simulink model "Sim6_02_lim_current_open_close_line"  (R2019b)
settings: Solver=ode1  StartTime=0.0  StopTime=6  FixedStep=Time_Step  MaxStep=1e-4  RelTol=1e-3
undefined symbols (not defined in the file): L_1, L_2, R_1, R_2, Time_Step, Ug, VSC01_id0
libraries: powerlib x14, simulink x4, Control_Lib x4, Source_Lib x1
settings Model: Creator=Frederic_Colas  LastModifiedBy=fcolas
settings DataIOCC: ReturnWorkspaceOutputs=off
settings OptimizationCC: LifeSpan=inf
settings DebuggingCC: UnconnectedInputMsg=none  UnconnectedOutputMsg=none  UnconnectedLineMsg=none  SFExecutionAtInitializationDiag=none  ArithmeticOperatorsInVariantConditions=warning
settings HardwareCC: ProdBitPerSizeT=32  ProdBitPerPtrDiffT=32  ProdWordSize=32  ProdHWDeviceType=Specified
settings SFSimCC: SimUseLocalCustomCode=off  CustomCodeUndefinedFunction=UseInterfaceOnly
settings RTWCC: RTWUseLocalCustomCode=off
settings CodeAppCC: StateflowObjectComments=on
settings SimscapeCC: SimscapeNormalizeSystem=off

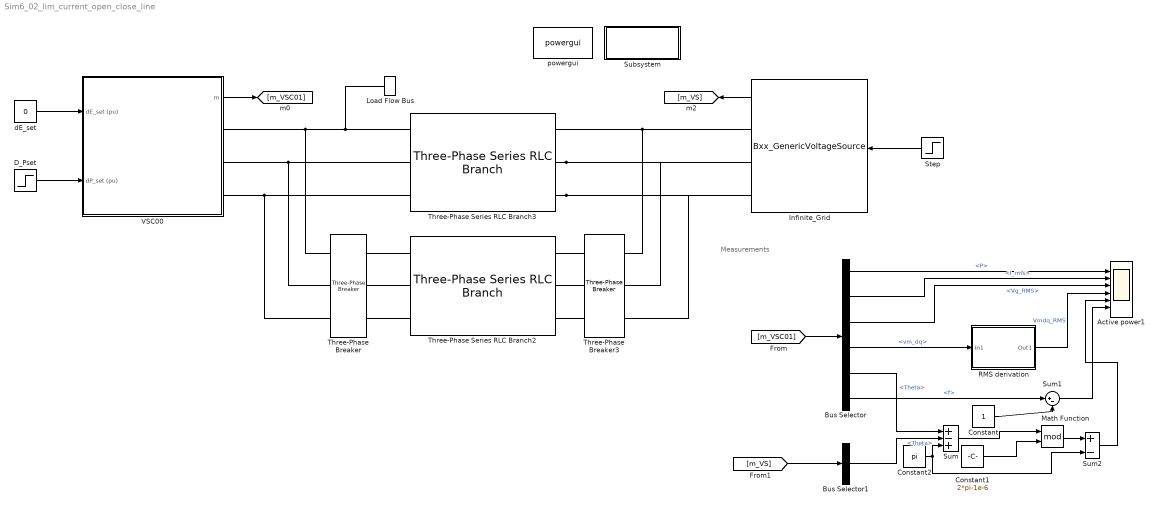
== system Sim6_02_lim_current_open_close_line ==
  note: Measurements
  Active power1 : Scope  NumInputPorts=6
  Bus Selector : BusSelector  OutputSignals=P,VI.I_rms,V.Vg_RMS,V.vm_dq,Theta.Theta,f
  Bus Selector1 : BusSelector  OutputSignals=Theta.Theta
  Constant : Constant
  Constant1 : Constant  Value=2*pi-1e-6
  Constant2 : Constant  Value=pi
  D_Pset : Step  After=0  SampleTime=0
  Infinite_Grid : Source_Lib/Bxx_GenericVoltageSource  SourceNature_str=INFINITE  fn=50  Sn=1e9  Un=Un  Time_Step=0  LFpopup=Swing  P0=-497498942.3663  Q0=24812063.8298  V0_pu=1  U0=20000  Theta0_deg=0  H_s=5  DroopOnOff=on  R_percent=4  TN=1  TD=2
      settings: SourceProductName=VSC4SPS
  Load Flow Bus : powerlib/Measurements/Load Flow Bus  LConnTagsString=a  Phases=single  Connectors=on one side  ID=BUS_1  Vbase=Un  Vref=1  Vangle=0  VLF=1.004  VLFb=1  VLFc=1  angleLF=2.855  angleLFb=0  angleLFc=0
  Math Function : Math  Operator=mod  SaturateOnIntegerOverflow=on
  RMS derivation : Subsystem
  Step : Step  Time=0.5  After=0  SampleTime=0
  Subsystem : Subsystem
      settings: OpenFcn=LoadFlow_VSC
      mask Display: color('blue'),disp('Update Loadflow')
  Sum : Sum  Inputs=+-+
  Sum1 : Sum  Inputs=|+-
  Sum2 : Sum  Inputs=+-
  Three-Phase Series RLC Branch2 : powerlib/Elements/Three-Phase Series RLC Branch  LConnTagsString=A|B|C  RConnTagsString=A|B|C  BranchType=RL  Resistance=R_2  Inductance=L_2  Capacitance=1e-6  Measurements=None
  Three-Phase Series RLC Branch3 : powerlib/Elements/Three-Phase Series RLC Branch  LConnTagsString=A|B|C  RConnTagsString=A|B|C  BranchType=RL  Resistance=R_1  Inductance=L_1  Capacitance=1e-6  Measurements=None
  Three-Phase Breaker : powerlib/Elements/Three-Phase Breaker  InitialState=closed  SwitchA=on  SwitchB=on  SwitchC=on  SwitchTimes=[1.5 4]  External=off  BreakerResistance=0.01  SnubberResistance=1e6  SnubberCapacitance=inf  Measurements=None
  Three-Phase Breaker3 : powerlib/Elements/Three-Phase Breaker  InitialState=closed  SwitchA=on  SwitchB=on  SwitchC=on  SwitchTimes=[1.5 4]  External=off  BreakerResistance=0.01  SnubberResistance=1e6  SnubberCapacitance=inf  Measurements=None
  VSC00 : Subsystem  mask(VSC){fn=50, Sn=1000e6, Pn=1000e6, Udcn=640e3, Time_Step=Time_Step, Un1=320e3, Un2=Ug, Rt_pu=0.005, Lt_pu=0.15, Lm_pu=500, Rm_pu=500, Tr_PLL=10, Val_Freq_Support=off, R_percent=4, Rv=0.09, W_TVR=60, I_max_VI_pu=1.2, DX_DR=5, Val_Mod_H=off, I_max_pu=1.25, Tr_I_max=200, Advanced=off, gainpopup=With Inertia, f_Inertia_Less=5/(2*pi), zeta_Inertia_Less=1, Param_Inertia=PI, H_GFo=5, zeta_GFo=0.7, LFpopup=PQ, P0=0.5, Q0=2.3716e-08, V0=1.0038, Theta0=2.8552}
      mask prompts: fn "Nominal Frequency (Hz)"; Sn "Nominal Apparent Power (VA)"; Pn "Nominal Power (W)"; Udcn "Nominal DC Voltage (V)"; Time_Step "Sample Time (s)"; Un1 "VSC side Nominal Ph-Ph Voltage (V)"; Un2 "Grid side Nominal Ph-Ph Voltage (V)"; Rt_pu "R (pu)"; Lt_pu "L (pu)"; Lm_pu "Rm (pu)"; Rm_pu "Lm (pu)"; Tr_PLL "Time response (ms)"; Val_Freq_Support "Frequency Support"; R_percent "Droop Gain (%)"; Rv "Damping Resistance (Rv)"; W_TVR "Dr filter"; I_max_VI_pu "Current Threshold (pu)"; Val_Mod_H "Inertia Modulation"; I_max_pu "I max (pu)"; Tr_I_max "Current Loop time response (ms)"; gainpopup "Strategy"; f_Inertia_Less "Bandwidth (Hz)"; zeta_Inertia_Less "Damping"; H_GFo "Inertia H (s)"; zeta_GFo "Damping Ratio"; P0 "Initial Active Power (pu)"; Q0 "Initial Reactive Power (pu)"; V0 "Initial Voltage (pu)"; Theta0 "Initial Angle (°)"
      mask init:
      | % Update Name of LF bus for internal purpose
      |     %NameStr = [get_param(gcb,'Name')];% '_LF'];
      |     %set_param([gcb '/Load Flow Bus'],'ID',NameStr);    
      |     
      | % Base values
      |     fb = fn;
      |     Pb = Pn;
      |     cos_phi_n = Pn/Sn;
      |     Sb = Pb/cos_phi_n;
      |     Vn1 = Un1/sqrt(3);
      |     Vb1 = Vn1;
      |     Vn2 = Un2/sqrt(3);
      |     Vb2 = Vn2;
      |     Ib1 = Sb / 3*Vb1;
      |     Ib2 = Sb / (3*Vb2);
      |     wb = 2*pi*fb;
      |   
      | % PLL derivation of the parameters
      |     wn_PLL=5/Tr_PLL;
      |     zeta_PLL = 1;
      |     Kp_PLL_pu = 2*zeta_PLL*wn_PLL/wb;
      |     Ki_PLL_pu = wn_PLL^2/wb;
      |     
      | % Grid-Forming control tuning
      |     % Inertia Less
      |     wn_Inertia_Less = 2*pi*f_Inertia_Less;
      |     Ki_Inertia_Less = Lt_pu*wn_Inertia_Less^2/wb;
      |     Kp_Inertia_Less = 2*zeta_Inertia_Less*wn_Inertia_Less*Lt_pu/wb;
      |     
      |     % With Inertia
      |     Kc = 1/(Lt_pu);
      |     kp_GFo = zeta_GFo*sqrt(2/(H_GFo*wb*Kc));
      |     kd = 2*H_GFo*kp_GFo*Kc*wb;
      | 
      | % Virtual Impedance tuning
      |     X_VI = roots([1/DX_DR^2+1 2*Lt_pu Lt_pu^2-1/I_max_VI_pu^2]);
      |     X_VI = max(X_VI);
      |     Kp_Rvi_pu = X_VI/(DX_DR*(I_max_VI_pu-1)); 
      |     
      | % Set the chosen strategy
      |     if (gainpopup == 1)
      |         Chosen_Strategy = 1;
      |     elseif (gainpopup == 2)
      |         if (Param_Inertia == 1)
      |             Chosen_Strategy = 2;
      |         elseif (Param_Inertia == 2)
      |             Chosen_Strategy = 3;
      |         end
      |     end
      |     
      | % Set the frequency droop gain
      |     R = R_percent / 100;
      | 
      | % Compute the delay compensation between control and power parts
      |     if (Time_Step == -1)
      |         Solver_Time_Step = 0;
      |     else
      |         Solver_Time_Step = Time_Step;
      |     end
      | 
      | % Compute Initial Voltage of VSC 
      | %   from steady-state output transformer model and Loadflow result
      |     
      |     %Initialize correctly the LoadFlow bus parameters connected to PCC
      |     VLF = V0;
      |     ThetaLF = Theta0;
      |     %if (LFpopup == 'PQ')
      |     %    VLF = 1;
      |     %    ThetaLF = 0;
      |     %elseif (LFpopup == 'PV')
      |     %%    VLF = V0;
      |     %    ThetaLF = 0;        
      |     %end
      |     %set_param([gcb '/Load Flow Bus'],'Vref',num2str(VLF),'Vangle',num2str(ThetaLF));
      |     
      |     R1_pu = Rt_pu/2;
      |     L1_pu = Lt_pu/2;
      |     R2_pu = Rt_pu/2;
      |     L2_pu = Lt_pu/2;
      |     X1_pu = L1_pu;
      |     X2_pu = L2_pu;
      |     Xm_pu = Lm_pu;
      |     
      |     Zm_pu = 1/(1/Rm_pu+1/(1i*Xm_pu));
      | 
      |     S0=P0+1i*Q0;
      |     I2 = conj(S0)/(V0);
      | 
      |     Vm = (R2_pu+1i*X2_pu)*I2 + V0;
      |     Im = Vm/Zm_pu;
      | 
      |     I1 = I2 + Im;
      |     V1 = (R1_pu+1i*X1_pu) * I1 + Vm;
      | 
      |     Vvsc0 = abs(V1);
      |     Theta_vsc0 = angle(V1) * 180/pi+Theta0;
      |     
      |     Va0 = Vvsc0*sqrt(2)*Vb1*sin(Theta_vsc0*pi/180);
      |     Vb0 = Vvsc0*sqrt(2)*Vb1*sin(Theta_vsc0*pi/180-2*pi/3);
      |     Vc0 = Vvsc0*sqrt(2)*Vb1*sin(Theta_vsc0*pi/180+2*pi/3);
      |     
      | % Generate string to display LF results on Mask
      |     %str_tmp = fprintf("Vvsc0 = %d, Theta_vsc0 = %d°",Vvsc0,Theta_vsc0);
      |     mo = get_param(gcb,'MaskObject');
      |     mo.getDialogControl('LF_vsc_str').Prompt = ['V0 = ', num2str(Vvsc0),' pu, Angle = ', num2str(Theta_vsc0),'°'];
      |     mo.getDialogControl('LF_pcc_str').Prompt = ['V0 = ', num2str(V0),' pu, Angle = ', num2str(Theta0),'°'];
      |     mo.getDialogControl('LF_pcc_Power_str').Prompt = ['P0 = ', num2str(P0),' pu, Q0 = ', num2str(Q0),' pu'];
      |     %set_param([gcb],'LF_str',str_tmp);
      settings: OpenFcn=|
      | NameStr = get_param(gcb,'Name');
      | open_system(gcbh, 'Mask');
      | 
      | h2AllOpenDlgs = DAStudio.ToolRoot.getOpenDialogs;
      | 
      | for i=1:length(h2AllOpenDlgs)
      |     try
      |          %disp(h2AllOpenDlgs(i).getSource.getBlock.Name);
      |         Dialog_block_name = h2AllOpenDlgs(i).getSource.getBlock.Name;
      |          %strcmp(Dialog_block_name, NameStr),
      |         if (strcmp(h2AllOpenDlgs(i).getSource.getBlock.Name, NameStr))
      |             iPos = h2AllOpenDlgs(i).position;
      |             h2AllOpenDlgs(i).position = [iPos(1)   iPos(2)   iPos(3)*1.4   iPos(4)];
      |         end
      |     end
      | end
      mask Callback Advanced:
      | % Get the mask parameter values. This is a cell
      | %   array of character vectors.
      | maskStr = get_param(gcb,'Advanced');
      | p=Simulink.Mask.get(gcb);
      | 
      | % The pop-up menu is the first mask parameter.
      | %   Check the value selected in the pop-up
      | if strcmp(maskStr,'on'),
      | 
      |     % Set the visibility of both parameters on when
      |     %   User-defined is selected in the pop-up.
      |     p.getDialogControl('TVR').Visible='on';
      |     p.getDialogControl('TVI').Visible='on';
      |     %p.getDialogControl('LC_Filter').Visible='on';
      |     p.getDialogControl('Current_Sat').Visible='on';
      |     %p.getDialogControl('Param_Strat_3').Visible='off';
      | 
      | 
      | else
      | 
      |     % Set the visibility of both parameters on when
      |     %   User-defined is selected in the pop-up.
      |     p.getDialogControl('TVR').Visible='off';
      |     p.getDialogControl('TVI').Visible='off';
      |     %p.getDialogControl('LC_Filter').Visible='off';
      |     p.getDialogControl('Current_Sat').Visible='off';
      |     %p.getDialogControl('Param_Strat_3').Visible='off';
      | 
      | end
      mask TypeOptions gainpopup: Inertia Less | With Inertia
      mask Callback gainpopup:
      | % Get the mask parameter values. This is a cell
      | %   array of character vectors.
      | maskStr = get_param(gcb,'gainpopup');
      | p=Simulink.Mask.get(gcb);
      | 
      | % The pop-up menu is the first mask parameter.
      | %   Check the value selected in the pop-up
      | if strcmp(maskStr,'Inertia Less'),
      | 
      |     % Set the visibility of both parameters on when
      |     %   User-defined is selected in the pop-up.
      |     p.getDialogControl('No_Inertia').Visible='on';
      |     p.getDialogControl('Inertia').Visible='off';
      |     %p.getDialogControl('Param_Strat_3').Visible='off';
      | 
      | 
      | elseif strcmp(maskStr,'With Inertia'),
      | 
      |     % Set the visibility of both parameters on when
      |     %   User-defined is selected in the pop-up.
      |     p.getDialogControl('No_Inertia').Visible='off';
      |     p.getDialogControl('Inertia').Visible='on';
      |     %p.getDialogControl('Param_Strat_3').Visible='off';
      | 
      | 
      |     % Turn off the visibility of the Value field
      |     %   when User-defined is not selected.
      | 
      | else
      | 
      |     % Set the visibility of both parameters on when
      |     %   User-defined is selected in the pop-up.
      |     p.getDialogControl('No_Inertia').Visible='off';
      |     p.getDialogControl('Inertia').Visible='off';
      |     %p.getDialogControl('Param_Strat_3').Visible='off';
      | 
      | end
      mask TypeOptions Param_Inertia: VSM | PI
      mask TypeOptions LFpopup: Swing | PQ | PV
      mask Callback LFpopup:
      | % Get the mask parameter values. This is a cell
      | %   array of character vectors.
      | maskStr = get_param(gcb,'LFpopup');
      | p=Simulink.Mask.get(gcb);
      | 
      | % The pop-up menu is the first mask parameter.
      | %   Check the value selected in the pop-up
      | if strcmp(maskStr,'Swing'),
      | 
      |     % Set the visibility of both parameters on when
      |     %   User-defined is selected in the pop-up.
      |     p.getParameter('P0').Visible='off';
      |     p.getParameter('Q0').Visible='off';
      |     p.getParameter('V0').Visible='on';
      |     p.getParameter('Theta0').Visible='on';
      |     set_param([gcb '/Source_For_LF'],'BusType','swing');
      | 
      | elseif strcmp(maskStr,'PQ'),
      | 
      |     % Set the visibility of both parameters on when
      |     %   User-defined is selected in the pop-up.
      |     p.getParameter('P0').Visible='on';
      |     p.getParameter('Q0').Visible='on';
      |     p.getParameter('V0').Visible='off';
      |     p.getParameter('Theta0').Visible='off';
      |     set_param([gcb '/Source_For_LF'],'BusType','PQ');
      | 
      |     % Turn off the visibility of the Value field
      |     %   when User-defined is not selected.
      | else
      | 
      |     % Set the visibility of both parameters on when
      |     %   User-defined is selected in the pop-up.
      |     p.getParameter('P0').Visible='on';
      |     p.getParameter('Q0').Visible='off';
      |     p.getParameter('V0').Visible='on';
      |     p.getParameter('Theta0').Visible='off';
      |     set_param([gcb '/Source_For_LF'],'BusType','PV');
      | 
      | end
      mask DialogControl Nominal_Param Prompt: Nominal Value
      mask DialogControl Container20 Prompt: Passive Components
      mask DialogControl Control_Param Prompt: Control Parameter
      mask DialogControl Container13 Prompt: PLL
      mask DialogControl Container14 Prompt: Frequency Support
      mask DialogControl TVR Prompt: Transient Virtual Resistor
      mask DialogControl TVI Prompt: Virtual Impedance
      mask DialogControl Current_Sat Prompt: Current Limitation
      mask DialogControl Container18 Prompt: Control Strategy
      mask DialogControl LF_Param Prompt: Loadflow
      mask DialogControl Control4 Prompt: Initial Operating Point
      mask DialogControl Container24 Prompt: VSC side
      mask DialogControl LF_vsc_str Prompt: V0 = 1.0092 pu, Angle = 7.1095°
      mask DialogControl Container25 Prompt: PCC
      mask DialogControl LF_pcc_str Prompt: V0 = 1.0038 pu, Angle = 2.8552°
      mask DialogControl LF_pcc_Power_str Prompt: P0 = 0.5 pu, Q0 = 2.3716e-08 pu
      mask DialogControl UpdateLoadflow Prompt: Update Loadflow
      mask DialogControl UpdateLoadflow Callback: LoadFlow_VSC
      mask Display:
      | x1=0.05;
      | y1=0.2;
      | %
      | plot([0.5 0.5]+x1,[0.97,0.8]-y1)
      | plot([0.5 0.32]+x1,[0.80 0.71]-y1)
      | plot([0.32 0.32]+x1,[0.80 0.52]-y1)
      | plot([0.32 0.5]+x1,[0.62 0.52]-y1)
      | plot([0.5 0.5]+x1,[0.52 0.35]-y1)
      | plot([0.45 0.5 0.43]+x1,[0.59 0.52 0.51]-y1)
      | %
      | plot([0.28 0.28]+x1,[0.74 0.58]-y1)
      | plot([0.28 0.20]+x1,[0.66 0.66]-y1)
      | %
      | plot([0.5 0.63]+x1,[0.84 0.84]-y1)
      | plot([0.63 0.63]+x1,[0.84 0.72]-y1)
      | plot([0.63 0.59]+x1,[0.72 0.65]-y1)
      | plot([0.63 0.67]+x1,[0.72 0.65]-y1)
      | plot([0.59 0.67]+x1,[0.65 0.65]-y1)
      | plot([0.63 0.63]+x1,[0.65 0.47]-y1)
      | plot([0.5 0.63]+x1,[0.47 0.47]-y1)
      | plot([0.58 0.67]+x1,[0.72 0.72]-y1)
      | %
      | color('blue')
      | text(0.3,0.10,'L-Filter GFo')
      | port_label('input',1,'dE_set (pu)');
      | port_label('input',2,'dP_set (pu)');
      | port_label('output',1,'m');
      | port_label('rconn',1,'A');
      | port_label('rconn',2,'B');
      | port_label('rconn',3,'C');
  dE_set : Constant  Value=0
  powergui : powerlib/powergui  Priority=1  SimulationMode=Discrete  SampleTime=Time_Step  frequency=60  Iterations=50  frequencyindice=50  Pbase=1000000000  ErrMax=1e-6  UnitsV=kV  UnitsW=MW  buscounter=0  FunctionMessages=off  echomessages=off  EnableUseOfTLC=off  CurrentSourceSwitches=off  DisableSnubberDevices=off  DisableRonSwitches=off  DisableVfSwitches=off  DisplayEquations=off  AutomaticDiscreteSolvers=off  SolverType=Tustin/Backward Euler (TBE)  Interpol=off  ExternalGateDelay=off  methode=off  Ts=100  x0status=blocks  SPID=on  SwTol=0  HookPort=off  NonlinearTolerance=1e-4  nMaxIteration=100  ContinueOnMaxIteration=off  RestoreLinks=warning  ResistiveCurrentMeasurement=off  Frange=[0:2:500]  Ylog=off  Xlog=on  ShowGrid=off  save=off  variable=ZData  structure=0  ZoomFFT=off  StartTime=0.0  cycles=1  DisplayStyle=1  fundamental=60  FreqAxis=off  MaxFrequency=1000  frequencyindicesteady=1  RmsSteady=1  display=off
  wires:
  dE_set/1 -> VSC00/1(dE_set (pu))
  D_Pset/1 -> VSC00/2(dP_set (pu))
  VSC00/1(m) -> [m_VSC01]
  Infinite_Grid/1 -> [m_VS]
  Step/1 -> Infinite_Grid/1
  Bus Selector/5 -> Sum/1  "<Theta>"
  Bus Selector/2 -> Active power1/2  "<I_rms>"
  RMS derivation/1(Out1) -> Active power1/4  "Vmdq_RMS"
  Sum1/1 -> Active power1/6
  Sum/1 -> Math Function/1
  Bus Selector/4 -> RMS derivation/1(In1)  "<vm_dq>"
  Bus Selector/6 -> Sum1/1  "<f>"
  Bus Selector1/1 -> Sum/2  "<Theta>"
  [m_VS] -> Bus Selector1/1
  Bus Selector/1 -> Active power1/1  "<P>"
  [m_VSC01] -> Bus Selector/1
  Bus Selector/3 -> Active power1/3  "<Vg_RMS>"
  Constant/1 -> Sum1/2
  Constant1/1 -> Math Function/2
  Math Function/1 -> Sum2/1
  Sum2/1 -> Active power1/5
  Constant2/1 -> Sum/3, Sum2/2
  connections:
  Three-Phase Breaker/LConn1 -- Three-Phase Series RLC Branch3/LConn1 -- Load Flow Bus/LConn1 -- VSC00/RConn1
  Three-Phase Series RLC Branch3/LConn3 -- VSC00/RConn3 -- Three-Phase Breaker/LConn3
  Three-Phase Series RLC Branch2/LConn2 -- Three-Phase Breaker/RConn2
  Three-Phase Series RLC Branch3/LConn2 -- VSC00/RConn2 -- Three-Phase Breaker/LConn2
  Three-Phase Series RLC Branch3/RConn2 -- Infinite_Grid/RConn2 -- Three-Phase Breaker3/RConn2
  Three-Phase Series RLC Branch2/LConn1 -- Three-Phase Breaker/RConn1
  Three-Phase Series RLC Branch2/LConn3 -- Three-Phase Breaker/RConn3
  Three-Phase Series RLC Branch3/RConn3 -- Infinite_Grid/RConn3 -- Three-Phase Breaker3/RConn3
  Three-Phase Series RLC Branch2/RConn1 -- Three-Phase Breaker3/LConn1
  Three-Phase Series RLC Branch2/RConn3 -- Three-Phase Breaker3/LConn3
  Three-Phase Series RLC Branch2/RConn2 -- Three-Phase Breaker3/LConn2
  Three-Phase Series RLC Branch3/RConn1 -- Three-Phase Breaker3/RConn1 -- Infinite_Grid/RConn1

== system Sim6_02_lim_current_open_close_line/RMS derivation ==
  In1 : Inport
  Demux : Demux  Outputs=2
  Sqrt : Sqrt  SaturateOnIntegerOverflow=on
  Square : Math  Operator=square  SaturateOnIntegerOverflow=on
  Square1 : Math  Operator=square  SaturateOnIntegerOverflow=on
  Sum : Sum
  Out1 : Outport
  wires:
  Square1/1 -> Sum/2
  Sum/1 -> Sqrt/1
  Sqrt/1 -> Out1/1
  Demux/1 -> Square/1
  Square/1 -> Sum/1
  Demux/2 -> Square1/1
  In1/1 -> Demux/1

== system Sim6_02_lim_current_open_close_line/Subsystem ==

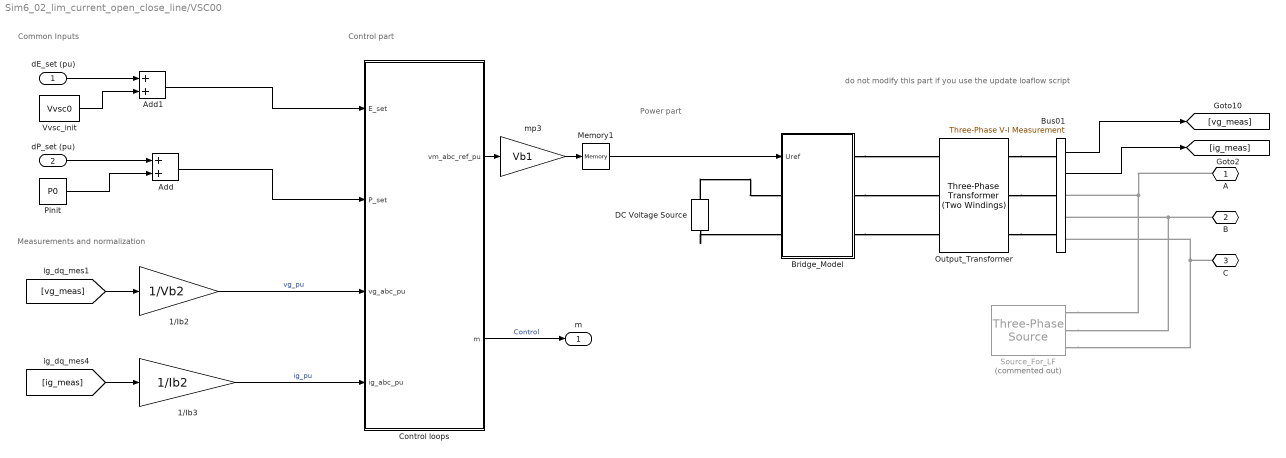
== system Sim6_02_lim_current_open_close_line/VSC00 ==
  note: do not modify this part if you use the update loaflow script
  note: Common Inputs
  note: Power part
  note: Measurements and normalization
  note: Control part
  dE_set (pu) : Inport
  dP_set (pu) : Inport  Port=2
  1/Ib2 : Gain  Gain=1/Vb2
  1/Ib3 : Gain  Gain=1/Ib2
  Add : Sum
  Add1 : Sum
  Bridge_Model : Subsystem
  Bus01 : powerlib/Measurements/Three-Phase V-I Measurement  VoltageMeasurement=phase-to-ground  SetLabelV=off  LabelV=Vabc  Vpu=off  VpuLL=off  CurrentMeasurement=yes  SetLabelI=off  LabelI=Iabc  Ipu=off  Pbase=100e6  Vbase=500e3  OutputType=Complex  PhasorSimulation=off  PSBequivalent=0
  Control loops : Subsystem
  DC Voltage Source : powerlib/Electrical Sources/DC Voltage Source  Amplitude=Udcn  Measurements=Voltage
  Memory1 : Memory  InitialCondition=[Va0 Vb0 Vc0]
  Output_Transformer : powerlib/Elements/Three-Phase Transformer (Two Windings)  Winding1Connection=Yg  Winding2Connection=Yg  CoreType=Three single-phase transformers  SetSaturation=off  Hysteresis=off  DataFile='hysteresis'  SetInitialFlux=off  Measurements=None  UNITS=pu  NominalPower=[Sn , fb]  Winding1=[Un1 , Rt_pu/2 , Lt_pu/2]  Winding2=[Un2 , Rt_pu/2 , Lt_pu/2]  Rm=Rm_pu  Lm=Lm_pu  L0=0.5  Saturation=[ 0,0 ; 0.0024,1.2 ; 1.0,1.52 ]  InitialFluxes=[ 0.8 , -0.8 , 0.7 ]  BreakLoop=off  DiscreteSolver=Trapezoidal iterative  DataType=off  TransfoNumber=1
  Pinit : Constant  Value=P0
  Source_For_LF : powerlib/Electrical Sources/Three-Phase Source  Commented=on  InternalConnection=Yg  VoltagePhases=off  Voltage=(400000)*1.00378  PhaseAngle=2.8552  Voltage_phases=[25e3 25e3 25e3]/sqrt(3)  PhaseAngles_phases=[0 -120 +120]  Frequency=fb  NonIdealSource=off  SpecifyImpedance=off  Resistance=0  Inductance=0  ShortCircuitLevel=100e6  BaseVoltage=Un  XRratio=7  BusType=PQ  Pref=P0*Sb  Qref=Q0*Sb  Prefabc=[10e3, 10e3, 10e3]  Qrefabc=[0, 0, 0]  Qmin=-inf  Qmax=inf
  Vvsc_init : Constant  Value=Vvsc0
  mp3 : Gain  Gain=Vb1
  A : PMIOPort  Side=Right
  B : PMIOPort  Port=2  Side=Right
  C : PMIOPort  Port=3  Side=Right
  m : Outport  VectorParamsAs1DForOutWhenUnconnected=off
  wires:
  Add/1 -> Control loops/2(P_set)
  Control loops/2(m) -> m/1  "Control"
  mp3/1 -> Memory1/1
  1/Ib3/1 -> Control loops/4(ig_abc_pu)  "ig_pu"
  1/Ib2/1 -> Control loops/3(vg_abc_pu)  "vg_pu"
  [vg_meas] -> 1/Ib2/1
  Control loops/1(vm_abc_ref_pu) -> mp3/1
  Add1/1 -> Control loops/1(E_set)
  Memory1/1 -> Bridge_Model/1(Uref)
  dP_set (pu)/1 -> Add/1
  Pinit/1 -> Add/2
  Vvsc_init/1 -> Add1/2
  Bus01/1 -> [vg_meas]
  dE_set (pu)/1 -> Add1/1
  Bus01/2 -> [ig_meas]
  [ig_meas] -> 1/Ib3/1
  connections:
  DC Voltage Source/LConn1 -- Bridge_Model/LConn2
  Output_Transformer/RConn1 -- Bus01/LConn1
  Output_Transformer/RConn2 -- Bus01/LConn2
  DC Voltage Source/RConn1 -- Bridge_Model/LConn1
  Output_Transformer/RConn3 -- Bus01/LConn3
  Source_For_LF/RConn2 -- B/RConn1 -- Bus01/RConn2
  Bridge_Model/RConn1 -- Output_Transformer/LConn1
  Bridge_Model/RConn2 -- Output_Transformer/LConn2
  Bridge_Model/RConn3 -- Output_Transformer/LConn3
  Source_For_LF/RConn1 -- A/RConn1 -- Bus01/RConn1
  Source_For_LF/RConn3 -- C/RConn1 -- Bus01/RConn3

== system Sim6_02_lim_current_open_close_line/VSC00/Bridge_Model ==
  Uref : Inport
  Constant : Constant
  Memory : Memory
  NOT1 : Logic  Operator=NOT  IconShape=distinctive  AllPortsSameDT=off  OutDataTypeStr=boolean
  Saturation : Saturate  UpperLimit=1  LowerLimit=-1
  Three-Phase Breaker1 : powerlib/Elements/Three-Phase Breaker  InitialState=closed  SwitchA=on  SwitchB=on  SwitchC=on  SwitchTimes="[4/60  10/60]"  External=on  BreakerResistance=0.001  SnubberResistance=1e6  SnubberCapacitance=inf  Measurements=None
  Three-Phase Breaker2 : powerlib/Elements/Three-Phase Breaker  InitialState=open  SwitchA=on  SwitchB=on  SwitchC=on  SwitchTimes="[4/60  10/60]"  External=on  BreakerResistance=0.001  SnubberResistance=1e6  SnubberCapacitance=inf  Measurements=None
  Three-Phase Source : powerlib/Electrical Sources/Three-Phase Source  InternalConnection=Yg  VoltagePhases=off  Voltage=Vvsc0*Un1  PhaseAngle=Theta_vsc0  Voltage_phases=[25e3 25e3 25e3]/sqrt(3)  PhaseAngles_phases=[0 -120 +120]  Frequency=fb  NonIdealSource=off  SpecifyImpedance=off  Resistance=0  Inductance=0  ShortCircuitLevel=100e6  BaseVoltage=VSC01_Un1  XRratio=7  BusType=swing  Pref=0.3  Qref=0  Prefabc=[10e3, 10e3, 10e3]  Qrefabc=[0, 0, 0]  Qmin=-Inf  Qmax=Inf
  Universal Bridge : powerlib/Power Electronics/Universal Bridge  Arms=3  SnubberResistance=1e5  SnubberCapacitance=inf  Device=Average-model based VSC  Ron=1e-3  Lon=0  ForwardVoltages="[  0  0  ]"  ForwardVoltage=0  GTOparameters=[ 10e-6 , 20e-6 ]  IGBTparameters=[ 1e-6 , 2e-6 ]  Measurements=None  Measurements_2=None  converterType=Rectifier
  mp3 : Gain  Gain=2/Udcn
  PhA : PMIOPort  Side=Right
  PhB : PMIOPort  Port=2  Side=Right
  PhC : PMIOPort  Port=3  Side=Right
  Vdc+ : PMIOPort  Port=4  Side=Left
  Vdc- : PMIOPort  Port=5  Side=Left
  wires:
  Saturation/1 -> Universal Bridge/1
  Constant/1 -> Memory/1
  NOT1/1 -> Three-Phase Breaker1/1
  Memory/1 -> NOT1/1, Three-Phase Breaker2/1
  mp3/1 -> Saturation/1
  Uref/1 -> mp3/1
  connections:
  Three-Phase Breaker2/LConn1 -- Three-Phase Breaker1/LConn1 -- PhA/RConn1
  Three-Phase Breaker2/LConn2 -- Three-Phase Breaker1/LConn2 -- PhB/RConn1
  Three-Phase Breaker2/LConn3 -- Three-Phase Breaker1/LConn3 -- PhC/RConn1
  Three-Phase Breaker2/RConn1 -- Universal Bridge/LConn1
  Three-Phase Breaker2/RConn2 -- Universal Bridge/LConn2
  Three-Phase Breaker2/RConn3 -- Universal Bridge/LConn3
  Three-Phase Source/RConn1 -- Three-Phase Breaker1/RConn1
  Three-Phase Source/RConn2 -- Three-Phase Breaker1/RConn2
  Three-Phase Source/RConn3 -- Three-Phase Breaker1/RConn3
  Universal Bridge/RConn1 -- Vdc+/RConn1
  Universal Bridge/RConn2 -- Vdc-/RConn1

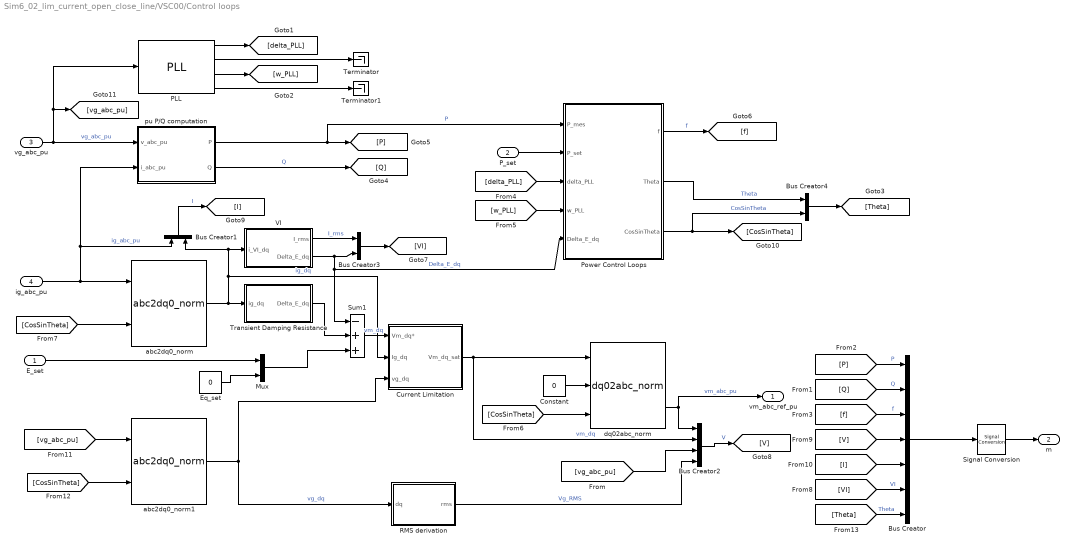
== system Sim6_02_lim_current_open_close_line/VSC00/Control loops ==
  E_set : Inport
  P_set : Inport  Port=2
  vg_abc_pu : Inport  Port=3
  ig_abc_pu : Inport  Port=4
  " pu P/Q computation" : Subsystem  DialogController=POWERSYS.PowerSysDialog
  Bus Creator : BusCreator  Inputs=7
  Bus Creator1 : BusCreator  Inputs=2
  Bus Creator2 : BusCreator  Inputs=4
  Bus Creator3 : BusCreator  Inputs=2
  Bus Creator4 : BusCreator  Inputs=2
  Constant : Constant  Value=0
  Current Limitation : Subsystem
  Eq_set : Constant  Value=0
  Mux : Mux  Inputs=2
  PLL : Control_Lib/PLL  fb=fb  Tr_PLL=Tr_PLL  Theta0=Theta0
      settings: SourceProductName=VSC_Lib
  Power Control Loops : Subsystem
  RMS derivation : Subsystem
  Signal Conversion : SignalConversion  OverrideOpt=off
  Sum1 : Sum  Inputs=-++
  Terminator : Terminator
  Terminator1 : Terminator
  Transient Damping Resistance : Subsystem
  VI : Subsystem
  abc2dq0_norm : Control_Lib/abc2dq0_norm  referenceAxisMode=Reference axis at 90 degrees behind phase_a  baseUpdateGain=1/sqrt(3)
      settings: SourceProductName=VSC_Lib
  abc2dq0_norm1 : Control_Lib/abc2dq0_norm  referenceAxisMode=Reference axis at 90 degrees behind phase_a  baseUpdateGain=1/sqrt(3)
      settings: SourceProductName=VSC_Lib
  dq02abc_norm : Control_Lib/dq02abc_norm  referenceAxisMode=Reference axis at 90 degrees behind phase_a  baseUpdateGain=sqrt(3)
      settings: SourceProductName=VSC_Lib
  vm_abc_ref_pu : Outport  VectorParamsAs1DForOutWhenUnconnected=off
  m : Outport  Port=2  VectorParamsAs1DForOutWhenUnconnected=off
  wires:
  [Theta] -> Bus Creator/7  "Theta"
  Bus Creator4/1 -> [Theta]
  RMS derivation/1(rms) -> Bus Creator2/4  "Vg_RMS"
  [vg_abc_pu] -> Bus Creator2/3
  Bus Creator3/1 -> [VI]
  PLL/4 -> Terminator1/1
  PLL/2 -> Terminator/1
  PLL/1 -> [delta_PLL]
  Constant/1 -> dq02abc_norm/2
  Power Control Loops/3(CosSinTheta) -> [CosSinTheta], Bus Creator4/2  "CosSinTheta"
  PLL/3 -> [w_PLL]
  [I] -> Bus Creator/5
  Bus Creator1/1 -> [I]  "I"
  Bus Creator/1 -> Signal Conversion/1
  [VI] -> Bus Creator/6  "VI"
  [V] -> Bus Creator/4
  Bus Creator2/1 -> [V]  "V"
  Eq_set/1 -> Mux/2
  Mux/1 -> Sum1/3
  VI/1(I_rms) -> Bus Creator3/1  "I_rms"
  Transient Damping Resistance/1("Delta_E_dq ") -> Sum1/2
  VI/2(Delta_E_dq) -> Bus Creator3/2, Sum1/1, Power Control Loops/5(Delta_E_dq)  "Delta_E_dq"
  [CosSinTheta] -> abc2dq0_norm/2
  [CosSinTheta] -> dq02abc_norm/3
  Power Control Loops/2(Theta) -> Bus Creator4/1  "Theta"
  abc2dq0_norm/2 -> Bus Creator1/2, VI/1(i_VI_dq), Current Limitation/2(Ig_dq), Transient Damping Resistance/1(ig_dq)  "ig_dq"
  ig_abc_pu/1 -> abc2dq0_norm/1, " pu P/Q computation"/2(i_abc_pu), Bus Creator1/1  "ig_abc_pu"
  " pu P/Q computation"/1(P) -> [P], Power Control Loops/1(P_mes)  "P"
  vg_abc_pu/1 -> PLL/1, [vg_abc_pu], " pu P/Q computation"/1(v_abc_pu)  "vg_abc_pu"
  Power Control Loops/1(f) -> [f]  "f"
  [w_PLL] -> Power Control Loops/4(w_PLL)
  P_set/1 -> Power Control Loops/2(P_set)
  [delta_PLL] -> Power Control Loops/3(delta_PLL)
  Current Limitation/1(Vm_dq_sat) -> dq02abc_norm/1, Bus Creator2/2  "vm_dq"
  " pu P/Q computation"/2(Q) -> [Q]  "Q"
  E_set/1 -> Mux/1
  dq02abc_norm/2 -> Bus Creator2/1, vm_abc_ref_pu/1  "vm_abc_pu"
  [f] -> Bus Creator/3  "f"
  [Q] -> Bus Creator/2  "Q"
  [P] -> Bus Creator/1  "P"
  Signal Conversion/1 -> m/1
  Sum1/1 -> Current Limitation/1(Vm_dq*)  "vm_dq"
  [vg_abc_pu] -> abc2dq0_norm1/1
  [CosSinTheta] -> abc2dq0_norm1/2
  abc2dq0_norm1/2 -> Current Limitation/3(vg_dq), RMS derivation/1(dq)  "vg_dq"

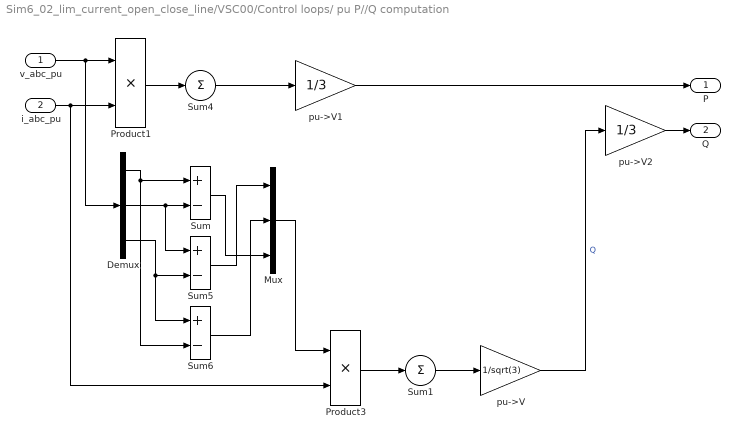
== system Sim6_02_lim_current_open_close_line/VSC00/Control loops/ pu P//Q computation ==
  v_abc_pu : Inport  PortDimensions=3
  i_abc_pu : Inport  Port=2  PortDimensions=3
  Demux : Demux  Outputs=3
      settings: DisplayOption=none
  Mux : Mux  Inputs=3
  Product1 : Product  InputSameDT=on  SaturateOnIntegerOverflow=on  OutDataTypeStr=Inherit: Same as first input
  Product3 : Product  InputSameDT=on  SaturateOnIntegerOverflow=on  OutDataTypeStr=Inherit: Same as first input
  Sum : Sum  Inputs=+-  InputSameDT=on  SaturateOnIntegerOverflow=on  OutDataTypeStr=Inherit: Same as first input
  Sum1 : Sum  Inputs=1  InputSameDT=on  SaturateOnIntegerOverflow=on  OutDataTypeStr=Inherit: Same as first input
  Sum4 : Sum  Inputs=1  InputSameDT=on  SaturateOnIntegerOverflow=on  OutDataTypeStr=Inherit: Same as first input
  Sum5 : Sum  Inputs=+-  InputSameDT=on  SaturateOnIntegerOverflow=on  OutDataTypeStr=Inherit: Same as first input
  Sum6 : Sum  Inputs=+-  InputSameDT=on  SaturateOnIntegerOverflow=on  OutDataTypeStr=Inherit: Same as first input
  pu->V : Gain  Gain=1/sqrt(3)  SaturateOnIntegerOverflow=on  OutDataTypeStr=Inherit: Same as input  ParamDataTypeStr=Inherit: Same as input
  pu->V1 : Gain  Gain=1/3  SaturateOnIntegerOverflow=on  OutDataTypeStr=Inherit: Same as input  ParamDataTypeStr=Inherit: Same as input
  pu->V2 : Gain  Gain=1/3  SaturateOnIntegerOverflow=on  OutDataTypeStr=Inherit: Same as input  ParamDataTypeStr=Inherit: Same as input
  P : Outport  VectorParamsAs1DForOutWhenUnconnected=off
  Q : Outport  Port=2  VectorParamsAs1DForOutWhenUnconnected=off
  wires:
  pu->V2/1 -> Q/1
  pu->V1/1 -> P/1
  Sum1/1 -> pu->V/1
  Product3/1 -> Sum1/1
  Product1/1 -> Sum4/1
  v_abc_pu/1 -> Product1/1, Demux/1
  i_abc_pu/1 -> Product1/2, Product3/2
  Sum4/1 -> pu->V1/1
  Demux/1 -> Sum/1, Sum6/2
  Demux/2 -> Sum/2, Sum5/1
  Demux/3 -> Sum5/2, Sum6/1
  Sum/1 -> Mux/3
  Sum5/1 -> Mux/1
  Sum6/1 -> Mux/2
  Mux/1 -> Product3/1
  pu->V/1 -> pu->V2/1  "Q"

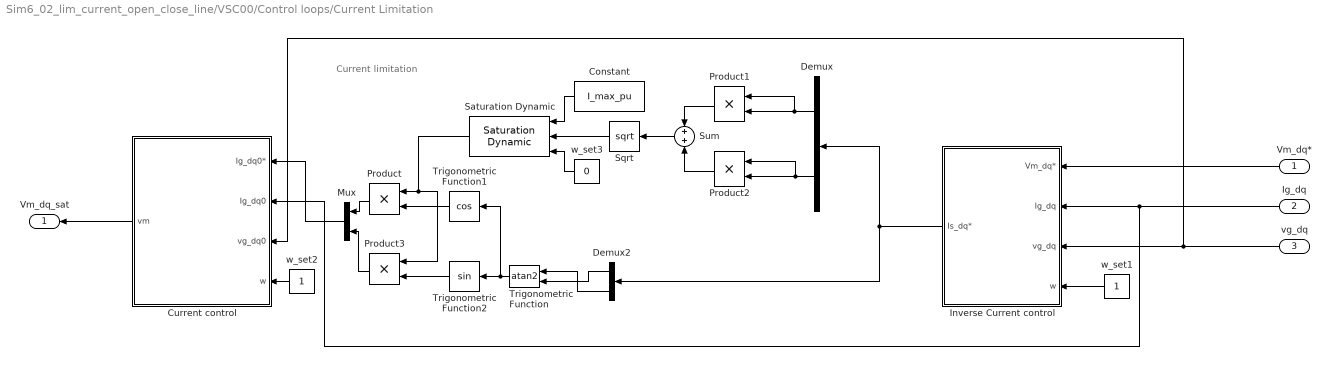
== system Sim6_02_lim_current_open_close_line/VSC00/Control loops/Current Limitation ==
  note: Current limitation
  Vm_dq* : Inport
  Ig_dq : Inport  Port=2
  vg_dq : Inport  Port=3
  Constant : Constant  Value=I_max_pu
  Current control : Subsystem
  Demux : Demux  Outputs=2
  Demux2 : Demux  Outputs=2
  Inverse Current control : Subsystem
  Mux : Mux  Inputs=2
  Product{,1..3} (4 alike) : Product
  Saturation Dynamic : simulink/Discontinuities/Saturation Dynamic  OutMin=[]  OutMax=[]  OutDataTypeStr=Inherit: Same as second input  OutDataType=fixdt(1, 16)  OutScaling=2^-10  DoSatur=off
  Sqrt : Sqrt  SaturateOnIntegerOverflow=on
  Sum : Sum
  Trigonometric Function : Trigonometry  Operator=atan2  NumberOfIterations=5  OutputSignalType=real
  Trigonometric Function1 : Trigonometry  Operator=cos
  Trigonometric Function2 : Trigonometry
  w_set1 : Constant
  w_set2 : Constant
  w_set3 : Constant  Value=0
  Vm_dq_sat : Outport  VectorParamsAs1DForOutWhenUnconnected=off
  wires:
  w_set3/1 -> Saturation Dynamic/3
  Constant/1 -> Saturation Dynamic/1
  Mux/1 -> Current control/1(Ig_dq0*)
  Product/1 -> Mux/1
  Demux/1 -> Product1/1, Product1/2
  Demux/2 -> Product2/1, Product2/2
  Trigonometric Function2/1 -> Product3/2
  Product2/1 -> Sum/2
  Trigonometric Function1/1 -> Product/2
  Demux2/1 -> Trigonometric Function/2
  Trigonometric Function/1 -> Trigonometric Function2/1, Trigonometric Function1/1
  Saturation Dynamic/1 -> Product/1, Product3/1
  Product1/1 -> Sum/1
  Sqrt/1 -> Saturation Dynamic/2
  Demux2/2 -> Trigonometric Function/1
  Inverse Current control/1(Is_dq*) -> Demux2/1, Demux/1
  Sum/1 -> Sqrt/1
  Product3/1 -> Mux/2
  Ig_dq/1 -> Inverse Current control/2(Ig_dq), Current control/2(Ig_dq0)
  w_set1/1 -> Inverse Current control/4(w)
  w_set2/1 -> Current control/4(w)
  vg_dq/1 -> Current control/3(vg_dq0), Inverse Current control/3(vg_dq)
  Vm_dq*/1 -> Inverse Current control/1(Vm_dq*)
  Current control/1(vm) -> Vm_dq_sat/1

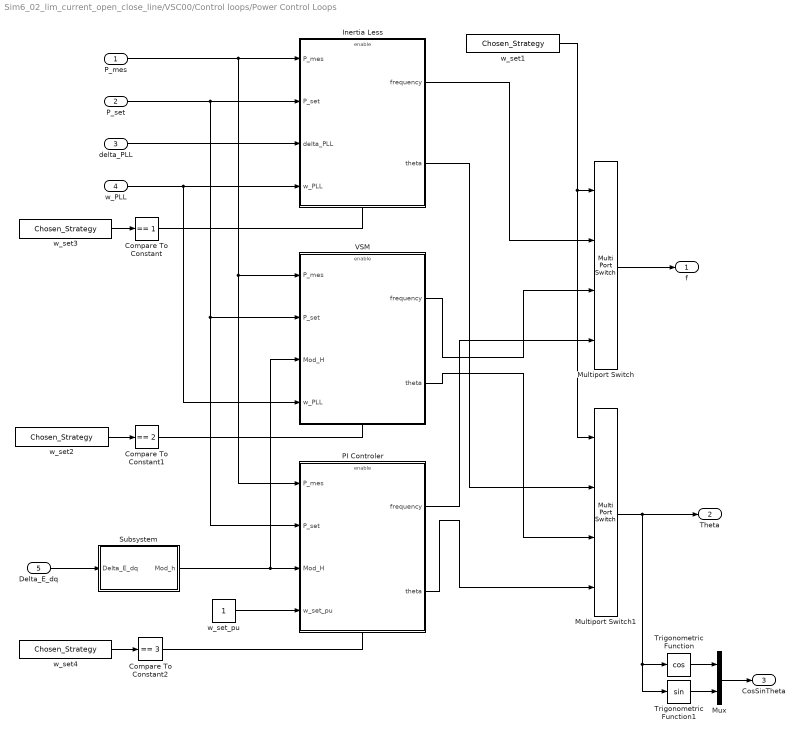
== system Sim6_02_lim_current_open_close_line/VSC00/Control loops/Power Control Loops ==
  P_mes : Inport
  P_set : Inport  Port=2
  delta_PLL : Inport  Port=3
  w_PLL : Inport  Port=4
  Delta_E_dq : Inport  Port=5
  Compare To Constant : simulink/Logic and Bit Operations/Compare To Constant  relop===  const=1  OutDataTypeStr=boolean
  Compare To Constant1 : simulink/Logic and Bit Operations/Compare To Constant  relop===  const=2  OutDataTypeStr=boolean
  Compare To Constant2 : simulink/Logic and Bit Operations/Compare To Constant  relop===  const=3  OutDataTypeStr=boolean
  Inertia Less : Subsystem
  Multiport Switch : MultiPortSwitch
  Multiport Switch1 : MultiPortSwitch
  Mux : Mux  Inputs=[1 1]
  PI Controler : Subsystem
  Subsystem : Subsystem
  Trigonometric Function : Trigonometry  Operator=cos
  Trigonometric Function1 : Trigonometry
  VSM : Subsystem
  w_set{1..4} (4 alike) : Constant  Value=Chosen_Strategy
  w_set_pu : Constant
  f : Outport  PortDimensions=1  VectorParamsAs1DForOutWhenUnconnected=off
  Theta : Outport  Port=2  VectorParamsAs1DForOutWhenUnconnected=off
  CosSinTheta : Outport  Port=3  PortDimensions=2  VectorParamsAs1DForOutWhenUnconnected=off
  wires:
  Subsystem/1(Mod_h) -> PI Controler/3(Mod_H), VSM/3(Mod_H)
  Delta_E_dq/1 -> Subsystem/1(Delta_E_dq)
  Multiport Switch1/1 -> Trigonometric Function1/1, Trigonometric Function/1, Theta/1
  Trigonometric Function1/1 -> Mux/2
  Mux/1 -> CosSinTheta/1
  Trigonometric Function/1 -> Mux/1
  Compare To Constant2/1 -> PI Controler/Enable
  Compare To Constant1/1 -> VSM/Enable
  Compare To Constant/1 -> Inertia Less/Enable
  w_set4/1 -> Compare To Constant2/1
  w_set2/1 -> Compare To Constant1/1
  w_set3/1 -> Compare To Constant/1
  Inertia Less/1(frequency) -> Multiport Switch/2
  Multiport Switch/1 -> f/1
  Inertia Less/2(theta) -> Multiport Switch1/2
  VSM/2(theta) -> Multiport Switch1/3
  w_set1/1 -> Multiport Switch/1, Multiport Switch1/1
  VSM/1(frequency) -> Multiport Switch/3
  PI Controler/1(frequency) -> Multiport Switch/4
  PI Controler/2(theta) -> Multiport Switch1/4
  w_set_pu/1 -> PI Controler/4(w_set_pu)
  w_PLL/1 -> Inertia Less/4(w_PLL), VSM/4(w_PLL)
  delta_PLL/1 -> Inertia Less/3(delta_PLL)
  P_set/1 -> Inertia Less/2(P_set), VSM/2(P_set), PI Controler/2(P_set)
  P_mes/1 -> Inertia Less/1(P_mes), VSM/1(P_mes), PI Controler/1(P_mes)

== system Sim6_02_lim_current_open_close_line/VSC00/Control loops/RMS derivation ==
  dq : Inport
  Demux : Demux  Outputs=2
  Sqrt : Sqrt  SaturateOnIntegerOverflow=on
  Square : Math  Operator=square  SaturateOnIntegerOverflow=on
  Square1 : Math  Operator=square  SaturateOnIntegerOverflow=on
  Sum : Sum
  rms : Outport
  wires:
  dq/1 -> Demux/1
  Demux/2 -> Square1/1
  Square/1 -> Sum/1
  Demux/1 -> Square/1
  Sqrt/1 -> rms/1
  Sum/1 -> Sqrt/1
  Square1/1 -> Sum/2

== system Sim6_02_lim_current_open_close_line/VSC00/Control loops/Transient Damping Resistance ==
  ig_dq : Inport
  Filter w_LF : Subsystem
      mask Display: disp('\omega_{LF} / (s + \omega_{LF})','texmode','on')
  Sum5 : Sum  Inputs=|+-
  nq1 : Gain  Gain=Rv
  "Delta_E_dq " : Outport  VectorParamsAs1DForOutWhenUnconnected=off
  wires:
  nq1/1 -> Filter w_LF/1(e), Sum5/2
  Filter w_LF/1(s) -> Sum5/1
  Sum5/1 -> "Delta_E_dq "/1
  ig_dq/1 -> nq1/1

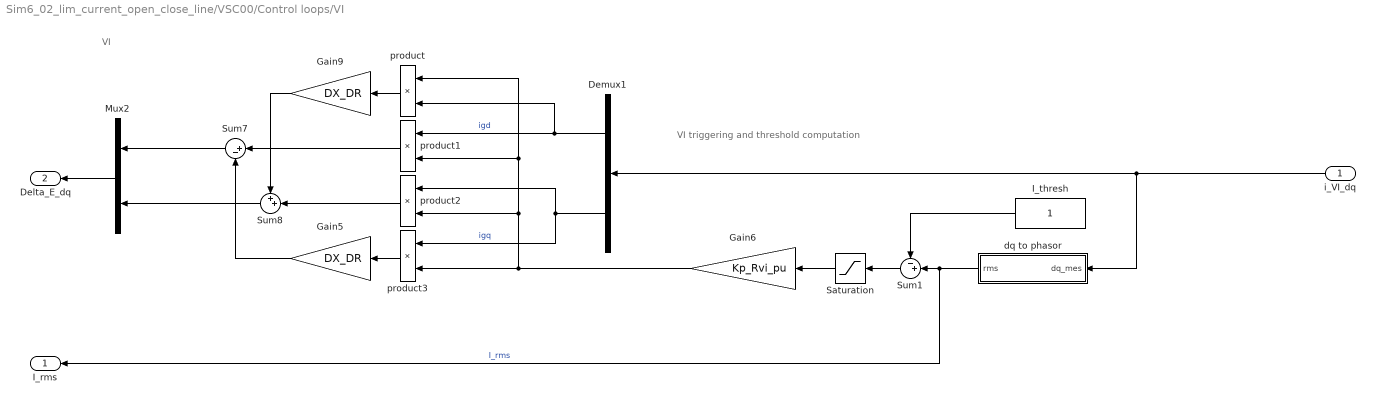
== system Sim6_02_lim_current_open_close_line/VSC00/Control loops/VI ==
  note: VI triggering and threshold computation
  note: VI
  i_VI_dq : Inport
  Demux1 : Demux  Outputs=2
      settings: DisplayOption=none
  Gain5 : Gain  Gain=DX_DR
  Gain6 : Gain  Gain=Kp_Rvi_pu
  Gain9 : Gain  Gain=DX_DR
  I_thresh : Constant
  Mux2 : Mux  Inputs=2
  Saturation : Saturate  UpperLimit=I_max_VI_pu-1  LowerLimit=0
  Sum1 : Sum  Inputs=-+|
  Sum7 : Sum  Inputs=|+-
  Sum8 : Sum  Inputs=++|
  dq to phasor : Subsystem
  product{,1..3} (4 alike) : Product  InputSameDT=on  RndMeth=Zero  SaturateOnIntegerOverflow=on  OutDataTypeStr=Inherit: Same as first input
  I_rms : Outport  VectorParamsAs1DForOutWhenUnconnected=off
  Delta_E_dq : Outport  Port=2  VectorParamsAs1DForOutWhenUnconnected=off
  wires:
  Sum1/1 -> Saturation/1
  dq to phasor/1(rms) -> Sum1/2, I_rms/1  "I_rms"
  Saturation/1 -> Gain6/1
  I_thresh/1 -> Sum1/1
  Mux2/1 -> Delta_E_dq/1
  Gain6/1 -> product3/2, product/1, product1/2, product2/2
  product3/1 -> Gain5/1
  product/1 -> Gain9/1
  Demux1/1 -> product1/1, product/2  "igd"
  Demux1/2 -> product2/1, product3/1  "igq"
  product1/1 -> Sum7/1
  Gain5/1 -> Sum7/2
  Gain9/1 -> Sum8/1
  product2/1 -> Sum8/2
  Sum7/1 -> Mux2/1
  Sum8/1 -> Mux2/2
  i_VI_dq/1 -> dq to phasor/1(dq_mes), Demux1/1

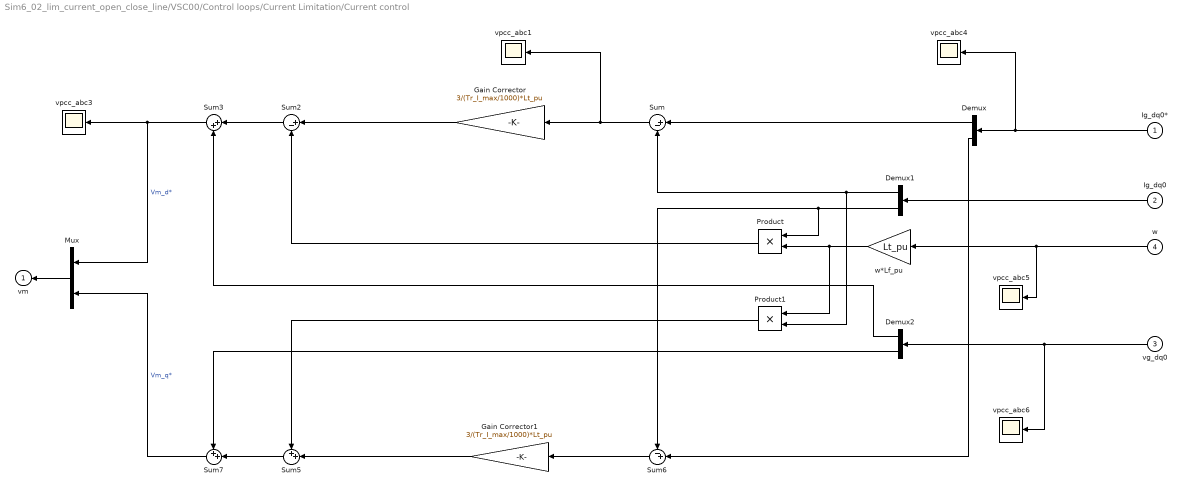
== system Sim6_02_lim_current_open_close_line/VSC00/Control loops/Current Limitation/Current control ==
  Ig_dq0* : Inport
  Ig_dq0 : Inport  Port=2
  vg_dq0 : Inport  Port=3
  w : Inport  Port=4
  Demux : Demux  Outputs=2
  Demux1 : Demux  Outputs=2
  Demux2 : Demux  Outputs=2
  Gain Corrector : Gain  Gain=3/(Tr_I_max/1000)*Lt_pu
  Gain Corrector1 : Gain  Gain=3/(Tr_I_max/1000)*Lt_pu
  Mux : Mux  Inputs=2
  Product : Product  RndMeth=Zero
  Product1 : Product  RndMeth=Zero
  Sum : Sum  Inputs=|+-
  Sum2 : Sum  Inputs=|+-
  Sum3 : Sum  Inputs=|++
  Sum5 : Sum  Inputs=++|
  Sum6 : Sum  Inputs=-+|
  Sum7 : Sum  Inputs=++|
  vpcc_abc{1,3..6} (5 alike) : Scope
  w*Lf_pu : Gain  Gain=Lt_pu
  vm : Outport  InitialOutput=0  VectorParamsAs1DForOutWhenUnconnected=off
  wires:
  Demux2/2 -> Sum7/1
  Demux2/1 -> Sum3/2
  w/1 -> vpcc_abc5/1, w*Lf_pu/1
  Sum/1 -> vpcc_abc1/1, Gain Corrector/1
  Sum7/1 -> Mux/2  "Vm_q*"
  Sum3/1 -> Mux/1, vpcc_abc3/1  "Vm_d*"
  Sum5/1 -> Sum7/2
  Product1/1 -> Sum5/1
  Gain Corrector1/1 -> Sum5/2
  Demux/2 -> Sum6/2
  Sum2/1 -> Sum3/1
  Product/1 -> Sum2/2
  Demux1/2 -> Sum6/1, Product/1
  w*Lf_pu/1 -> Product/2, Product1/1
  Gain Corrector/1 -> Sum2/1
  Demux1/1 -> Sum/2, Product1/2
  Demux/1 -> Sum/1
  Ig_dq0/1 -> Demux1/1
  vg_dq0/1 -> Demux2/1, vpcc_abc6/1
  Sum6/1 -> Gain Corrector1/1
  Ig_dq0*/1 -> vpcc_abc4/1, Demux/1
  Mux/1 -> vm/1

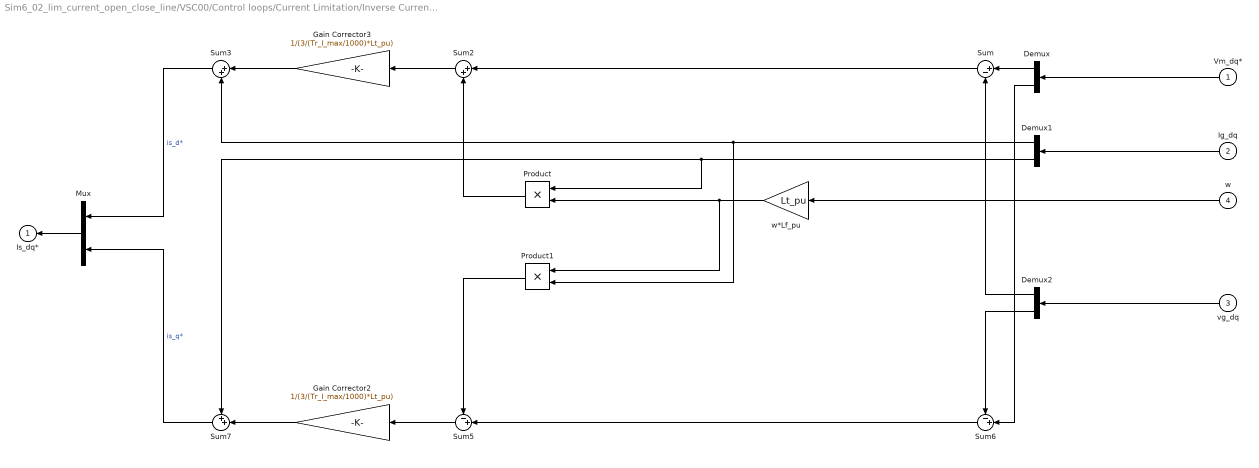
== system Sim6_02_lim_current_open_close_line/VSC00/Control loops/Current Limitation/Inverse Current control ==
  Vm_dq* : Inport
  Ig_dq : Inport  Port=2
  vg_dq : Inport  Port=3
  w : Inport  Port=4
  Demux : Demux  Outputs=2
  Demux1 : Demux  Outputs=2
  Demux2 : Demux  Outputs=2
  Gain Corrector2 : Gain  Gain=1/(3/(Tr_I_max/1000)*Lt_pu)
  Gain Corrector3 : Gain  Gain=1/(3/(Tr_I_max/1000)*Lt_pu)
  Mux : Mux  Inputs=2
  Product : Product  RndMeth=Zero
  Product1 : Product  RndMeth=Zero
  Sum : Sum  Inputs=|+-
  Sum2 : Sum  Inputs=|++
  Sum3 : Sum  Inputs=|++
  Sum5 : Sum  Inputs=-+|
  Sum6 : Sum  Inputs=-+|
  Sum7 : Sum  Inputs=++|
  w*Lf_pu : Gain  Gain=Lt_pu
  Is_dq* : Outport  InitialOutput=0  VectorParamsAs1DForOutWhenUnconnected=off
  wires:
  vg_dq/1 -> Demux2/1
  Ig_dq/1 -> Demux1/1
  Vm_dq*/1 -> Demux/1
  Demux/1 -> Sum/1
  Demux1/1 -> Sum3/2, Product1/2
  Sum/1 -> Sum2/1
  w*Lf_pu/1 -> Product1/1, Product/2
  Product/1 -> Sum2/2
  Sum2/1 -> Gain Corrector3/1
  Mux/1 -> Is_dq*/1
  Demux/2 -> Sum6/2
  Sum6/1 -> Sum5/2
  Sum5/1 -> Gain Corrector2/1
  Sum3/1 -> Mux/1  "is_d*"
  Sum7/1 -> Mux/2  "is_q*"
  w/1 -> w*Lf_pu/1
  Demux1/2 -> Sum7/1, Product/1
  Gain Corrector3/1 -> Sum3/1
  Demux2/1 -> Sum/2
  Demux2/2 -> Sum6/1
  Product1/1 -> Sum5/1
  Gain Corrector2/1 -> Sum7/2

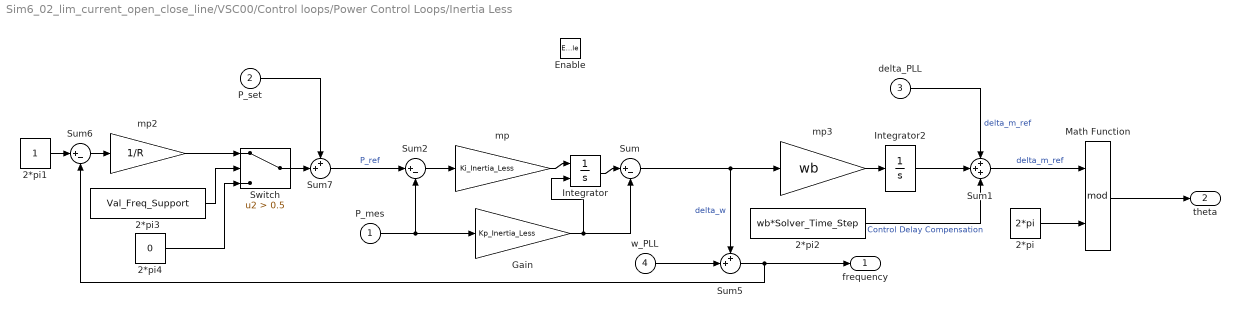
== system Sim6_02_lim_current_open_close_line/VSC00/Control loops/Power Control Loops/Inertia Less ==
  P_mes : Inport
  P_set : Inport  Port=2
  delta_PLL : Inport  Port=3
  w_PLL : Inport  Port=4
  Enable : EnablePort
  2*pi : Constant  Value=2*pi
  2*pi1 : Constant
  2*pi2 : Constant  Value=wb*Solver_Time_Step
  2*pi3 : Constant  Value=Val_Freq_Support
  2*pi4 : Constant  Value=0
  Gain : Gain  Gain=Kp_Inertia_Less
  Integrator : Integrator  InitialConditionSource=external
  Integrator2 : Integrator  InitialCondition=(Theta_vsc0)*pi/180-Theta0*pi/180
  Math Function : Math  Operator=mod  SignedPower=on  SaturateOnIntegerOverflow=on
  Sum : Sum  Inputs=|+-
  Sum1 : Sum  Inputs=+++
  Sum2 : Sum  Inputs=|+-
  Sum5 : Sum  Inputs=++|
  Sum6 : Sum  Inputs=|+-
  Sum7 : Sum  Inputs=++|
  Switch : Switch  Criteria=u2 > Threshold  Threshold=0.5
  mp : Gain  Gain=Ki_Inertia_Less
  mp2 : Gain  Gain=1/R
  mp3 : Gain  Gain=wb
  frequency : Outport  VectorParamsAs1DForOutWhenUnconnected=off
  theta : Outport  Port=2  VectorParamsAs1DForOutWhenUnconnected=off
  wires:
  Gain/1 -> Sum/2, Integrator/2
  Integrator/1 -> Sum/1
  2*pi4/1 -> Switch/3
  2*pi3/1 -> Switch/2
  mp2/1 -> Switch/1
  Integrator2/1 -> Sum1/2
  2*pi2/1 -> Sum1/3  "Control Delay Compensation"
  Sum5/1 -> Sum6/2, frequency/1
  w_PLL/1 -> Sum5/2
  delta_PLL/1 -> Sum1/1  "delta_m_ref"
  mp/1 -> Integrator/1
  mp3/1 -> Integrator2/1
  Sum/1 -> Sum5/1, mp3/1  "delta_w"
  Math Function/1 -> theta/1
  Switch/1 -> Sum7/2
  P_mes/1 -> Sum2/2, Gain/1
  Sum7/1 -> Sum2/1  "P_ref"
  P_set/1 -> Sum7/1
  Sum6/1 -> mp2/1
  2*pi1/1 -> Sum6/1
  2*pi/1 -> Math Function/2
  Sum1/1 -> Math Function/1  "delta_m_ref"
  Sum2/1 -> mp/1

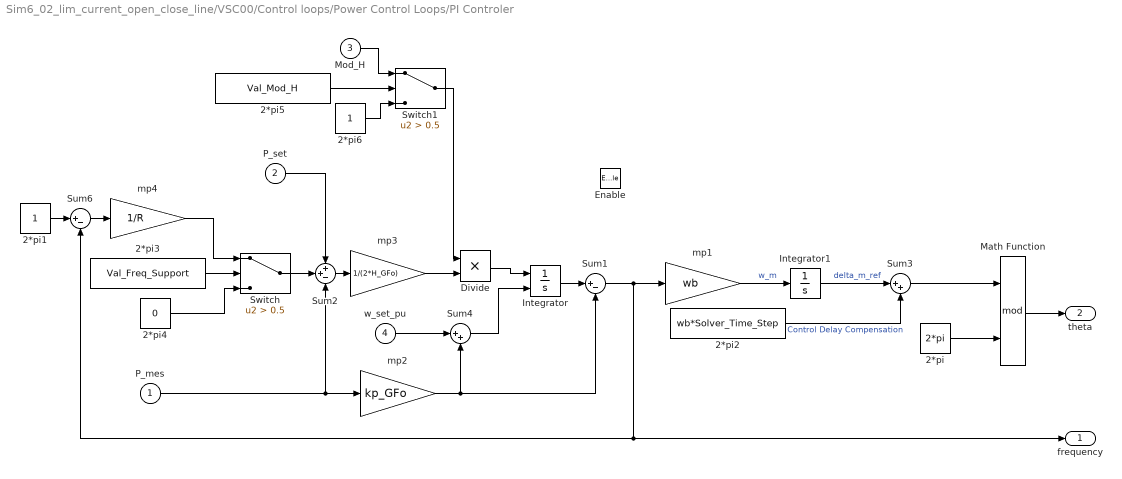
== system Sim6_02_lim_current_open_close_line/VSC00/Control loops/Power Control Loops/PI Controler ==
  P_mes : Inport
  P_set : Inport  Port=2
  Mod_H : Inport  Port=3
  w_set_pu : Inport  Port=4
  Enable : EnablePort
  2*pi : Constant  Value=2*pi
  2*pi1 : Constant
  2*pi2 : Constant  Value=wb*Solver_Time_Step
  2*pi3 : Constant  Value=Val_Freq_Support
  2*pi4 : Constant  Value=0
  2*pi5 : Constant  Value=Val_Mod_H
  2*pi6 : Constant
  Divide : Product  Inputs=**
  Integrator : Integrator  InitialConditionSource=external
  Integrator1 : Integrator  InitialCondition=(Theta_vsc0)*pi/180
  Math Function : Math  Operator=mod  SignedPower=on  SaturateOnIntegerOverflow=on
  Sum1 : Sum  Inputs=|+-
  Sum2 : Sum  Inputs=++-
  Sum3 : Sum  Inputs=|++
  Sum4 : Sum  Inputs=|++
  Sum6 : Sum  Inputs=|+-
  Switch : Switch  Criteria=u2 > Threshold  Threshold=0.5
  Switch1 : Switch  Criteria=u2 > Threshold  Threshold=0.5
  mp1 : Gain  Gain=wb
  mp2 : Gain  Gain=kp_GFo
  mp3 : Gain  Gain=1/(2*H_GFo)
  mp4 : Gain  Gain=1/R
  frequency : Outport  VectorParamsAs1DForOutWhenUnconnected=off
  theta : Outport  Port=2  VectorParamsAs1DForOutWhenUnconnected=off
  wires:
  Switch1/1 -> Divide/1
  Divide/1 -> Integrator/1
  Mod_H/1 -> Switch1/1
  2*pi6/1 -> Switch1/3
  2*pi5/1 -> Switch1/2
  Switch/1 -> Sum2/2
  2*pi4/1 -> Switch/3
  Sum6/1 -> mp4/1
  2*pi3/1 -> Switch/2
  2*pi1/1 -> Sum6/1
  mp4/1 -> Switch/1
  Sum4/1 -> Integrator/2
  mp3/1 -> Divide/2
  mp2/1 -> Sum4/2, Sum1/2
  P_mes/1 -> mp2/1, Sum2/3
  2*pi2/1 -> Sum3/2  "Control Delay Compensation"
  Sum3/1 -> Math Function/1
  mp1/1 -> Integrator1/1  "w_m"
  Sum1/1 -> Sum6/2, frequency/1, mp1/1
  Integrator/1 -> Sum1/1
  P_set/1 -> Sum2/1
  w_set_pu/1 -> Sum4/1
  2*pi/1 -> Math Function/2
  Math Function/1 -> theta/1
  Integrator1/1 -> Sum3/1  "delta_m_ref"
  Sum2/1 -> mp3/1

== system Sim6_02_lim_current_open_close_line/VSC00/Control loops/Power Control Loops/Subsystem ==
  Delta_E_dq : Inport
  Constant : Constant
  Constant1 : Constant  Value=2
  Delay : Delay  DelayLength=1  InitialCondition=1
  Demux : Demux  Outputs=2
  Pow : Math  Operator=pow  SignedPower=on  RndMeth=Zero  SaturateOnIntegerOverflow=on
  Square : Math  Operator=square  SignedPower=on  RndMeth=Zero  SaturateOnIntegerOverflow=on
  Square1 : Math  Operator=square  SignedPower=on  RndMeth=Zero  SaturateOnIntegerOverflow=on
  Sum : Sum  Inputs=|+-
  Sum5 : Sum
  Mod_h : Outport  VectorParamsAs1DForOutWhenUnconnected=off
  wires:
  Delay/1 -> Demux/1
  Sum/1 -> Square/1
  Demux/1 -> Sum/2
  Square1/1 -> Sum5/2
  Sum5/1 -> Pow/1
  Constant/1 -> Sum/1
  Demux/2 -> Square1/1
  Constant1/1 -> Pow/2
  Pow/1 -> Mod_h/1
  Square/1 -> Sum5/1
  Delta_E_dq/1 -> Delay/1

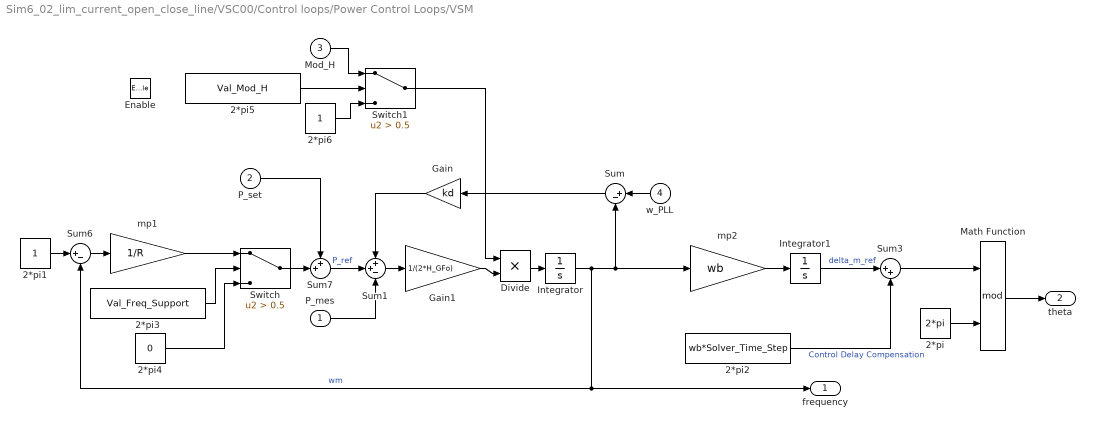
== system Sim6_02_lim_current_open_close_line/VSC00/Control loops/Power Control Loops/VSM ==
  P_mes : Inport
  P_set : Inport  Port=2
  Mod_H : Inport  Port=3
  w_PLL : Inport  Port=4
  Enable : EnablePort
  2*pi : Constant  Value=2*pi
  2*pi1 : Constant
  2*pi2 : Constant  Value=wb*Solver_Time_Step
  2*pi3 : Constant  Value=Val_Freq_Support
  2*pi4 : Constant  Value=0
  2*pi5 : Constant  Value=Val_Mod_H
  2*pi6 : Constant
  Divide : Product  Inputs=**
  Gain : Gain  Gain=kd
  Gain1 : Gain  Gain=1/(2*H_GFo)
  Integrator : Integrator  InitialCondition=1
  Integrator1 : Integrator  InitialCondition=Theta_vsc0*pi/180
  Math Function : Math  Operator=mod  SignedPower=on  SaturateOnIntegerOverflow=on
  Sum : Sum  Inputs=|+-
  Sum1 : Sum  Inputs=++-
  Sum3 : Sum  Inputs=|++
  Sum6 : Sum  Inputs=|+-
  Sum7 : Sum  Inputs=++|
  Switch : Switch  Criteria=u2 > Threshold  Threshold=0.5
  Switch1 : Switch  Criteria=u2 > Threshold  Threshold=0.5
  mp1 : Gain  Gain=1/R
  mp2 : Gain  Gain=wb
  frequency : Outport  VectorParamsAs1DForOutWhenUnconnected=off
  theta : Outport  Port=2  VectorParamsAs1DForOutWhenUnconnected=off
  wires:
  Switch1/1 -> Divide/1
  Gain1/1 -> Divide/2
  Divide/1 -> Integrator/1
  Mod_H/1 -> Switch1/1
  2*pi6/1 -> Switch1/3
  2*pi5/1 -> Switch1/2
  Sum7/1 -> Sum1/2  "P_ref"
  Sum1/1 -> Gain1/1
  Gain/1 -> Sum1/1
  Sum/1 -> Gain/1
  w_PLL/1 -> Sum/1
  2*pi4/1 -> Switch/3
  2*pi3/1 -> Switch/2
  mp1/1 -> Switch/1
  2*pi1/1 -> Sum6/1
  Sum6/1 -> mp1/1
  P_set/1 -> Sum7/1
  Switch/1 -> Sum7/2
  Sum3/1 -> Math Function/1
  2*pi2/1 -> Sum3/2  "Control Delay Compensation"
  mp2/1 -> Integrator1/1
  P_mes/1 -> Sum1/3
  Integrator/1 -> Sum6/2, frequency/1, mp2/1, Sum/2  "wm"
  Integrator1/1 -> Sum3/1  "delta_m_ref"
  Math Function/1 -> theta/1
  2*pi/1 -> Math Function/2

== system Sim6_02_lim_current_open_close_line/VSC00/Control loops/Transient Damping Resistance/Filter w_LF ==
  e : Inport
  1/T_LP : Gain  Gain=W_TVR  SaturateOnIntegerOverflow=on  OutDataTypeStr=Inherit: Same as input  ParamDataTypeStr=Inherit: Same as input
  Integrator : Integrator  InitialConditionSource=external  InitialCondition=[VSC01_id0*0.04]
  Sum1 : Sum  Inputs=|+-  InputSameDT=on  SaturateOnIntegerOverflow=on  OutDataTypeStr=Inherit: Same as first input
  s : Outport  VectorParamsAs1DForOutWhenUnconnected=off
  wires:
  e/1 -> Sum1/1, Integrator/2
  Integrator/1 -> s/1, Sum1/2
  1/T_LP/1 -> Integrator/1
  Sum1/1 -> 1/T_LP/1

== system Sim6_02_lim_current_open_close_line/VSC00/Control loops/VI/dq to phasor ==
  dq_mes : Inport
  Demux : Demux  Outputs=2
      settings: DisplayOption=none
  Sqrt : Sqrt  SaturateOnIntegerOverflow=on
  Sum4 : Sum  Inputs=|++  InputSameDT=on  SaturateOnIntegerOverflow=on  OutDataTypeStr=Inherit: Same as first input
  Vrdird : Product  InputSameDT=on  RndMeth=Zero  SaturateOnIntegerOverflow=on  OutDataTypeStr=Inherit: Same as first input
  Vrqirq : Product  InputSameDT=on  RndMeth=Zero  SaturateOnIntegerOverflow=on  OutDataTypeStr=Inherit: Same as first input
  rms : Outport  VectorParamsAs1DForOutWhenUnconnected=off
  wires:
  Sum4/1 -> Sqrt/1
  Vrqirq/1 -> Sum4/2
  Vrdird/1 -> Sum4/1
  Demux/2 -> Vrqirq/2, Vrqirq/1
  Demux/1 -> Vrdird/2, Vrdird/1
  dq_mes/1 -> Demux/1
  Sqrt/1 -> rms/1
